simulink library "cdma2000_lib"  (Simulink 6.0)
settings: Solver=ode45  SolverMode=SingleTasking  StartTime=0.0  StopTime=10.0  RelTol=1e-3
values from neighbouring files (symbols this model uses):
  numTapsChEst = str2num(Vals{idxNumTapsChEst})    [wcdma_initmaskphlayer.m]    (also in wcdma_initmaskspreadandmod.m; wcdma_loadinitphlayer.m = 21; wcdma_loadinitspreadandmod.m = 21)
  overSampling = str2num(Vals{idxOverSampling})    [wcdma_initmaskphlayer.m]    (also in wcdma_initmaskspreadandmod.m; wcdma_loadinitphlayer.m = 8; wcdma_loadinitspreadandmod.m = 8)
undefined symbols (not defined in the file or in its folder): decPattern, gateRate, j, longCodeScrOff, magnitude, numPuncturedSymbols, numSymbPCGroup, overSamp, PCGroupInit, plcm_37, powerControlOff, qof_sign, scrBitRepetition, symbolTime, walshLength
libraries: dspsigops x30, dspsrcs4 x29, commutil2 x14, cdma2000_lib x13, commseqgen2 x10, dspbuff3 x9, dspsigattribs x7, dspindex x5, commsequence2 x4, commchan2 x3, simulink x3, dspmtrx3 x2
(part 1 of 2)
settings Model: Creator=arodrigu  LastModifiedBy=arodrigu  ProdHWDeviceType=Specified
settings DataIOCC: SignalLoggingName=logsOut
settings OptimizationCC: BooleanDataType=off
settings DebuggingCC: CheckExecutionContextPreStartOutputMsg=on  CheckExecutionContextRuntimeOutputMsg=on  SolverPrmCheckMsg=none
settings HardwareCC: ProdHWDeviceType=Specified  TargetUnknown=on
settings ModelReferenceCC: UpdateModelReferenceTargets=IfOutOfDate
settings SFSimCC: SFSimApplyToAllLibs=on  SFSimBuildMode=Incremental

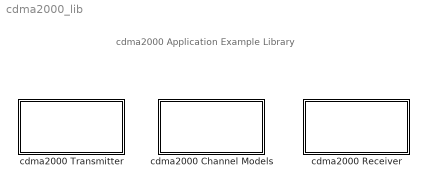
== system cdma2000_lib ==
  note: cdma2000 Application
      | Example Library
  cdma2000 Channel Models : Subsystem  PropExecContextAcrossSSBoundary=on
      mask Display: disp('cdma2000\nChannel Models')
  cdma2000 Receiver : Subsystem  PropExecContextAcrossSSBoundary=on
      mask Display: disp('cdma2000\nReceiver')
  cdma2000 Transmitter : Subsystem  PropExecContextAcrossSSBoundary=on
      mask Display: disp('cdma2000\nTransmitter')

== system cdma2000_lib/cdma2000 Channel Models ==
  note: cdma2000 Channel Models sublibrary
  AWGN Channel : Subsystem  PropExecContextAcrossSSBoundary=on  mask(cdma2000 Channel model: AWGN Channel){EsNodB=0}
      mask prompts: EsNodB "Es/No (dB):"
      mask Display: disp('AWGN Channel')
  Configurable Subsystem : Subsystem  BlockChoice=AWGN Channel  PropExecContextAcrossSSBoundary=on
      settings: TemplateBlock=self  MemberBlocks=AWGN Channel,Multipath Fading Channel,No Channel
  Multipath Fading Channel : Subsystem  PropExecContextAcrossSSBoundary=on  mask(cdma2000 Channel model: Multipath Fading Channel){EcN0=10, dopplerFreq=486, delayVector=[0 260e-9 521e-9 781e-9], gainVector=[0 -3 -6 -9]}
      mask prompts: EcN0 "EcN0 (in dB):"; dopplerFreq "Maximum Doppler Frequency shift (in Hz):"; delayVector "Multipath Profile - Delay Vector (s):"; gainVector "Multipath Profile - Gain Vector (dB):"
      mask Display: disp('Multipath Fading\nAWGN')
  No Channel : Subsystem  PropExecContextAcrossSSBoundary=on
      mask Type: cdma2000 Channel model: No Channel
      mask Display: disp('No Channel')

== system cdma2000_lib/cdma2000 Receiver ==
  note: cdma2000 Receiver sublibrary
  Channel Estimation : Subsystem  PropExecContextAcrossSSBoundary=on  mask(Channel Estimation){numTapsChEst=21}
      mask prompts: numTapsChEst "Number of Filter Taps for Channel Estimation:"
      mask help: Perform Channel Estimation
  Data Correlator : Subsystem  TreatAsAtomicUnit=on  PropExecContextAcrossSSBoundary=on
      mask Type: Data Correlator
  Long Code DeScrambling : Subsystem  PropExecContextAcrossSSBoundary=on
  Long Code DeScrambling Power Control Extracting : Subsystem  PropExecContextAcrossSSBoundary=on  mask(Long Code DeScrambling){radConfig=Radio Configuration 3, numSamp=768, nFrameMask=1, longCScrMask=Off, gateRateMask=1/4, TxDivMode=Non-TD, plcMask=[1 1 0 0 0 plcm_37]}
      mask prompts: radConfig "Radio Configuration:"; numSamp "Number of Samples per Frame:"; nFrameMask "Length of frame in multiples of 20 ms (n):"; longCScrMask "Long Code Scrambling"; gateRateMask "Gated Trasmission Rate:"; TxDivMode "Transmit Diversity Mode:"; plcMask "Public Long Code Mask:"
      mask help: Performs Long Code DeScrambling and Power Control Extraction for Forward Traffic Channel.
      mask init:
      | %-- Initialize parameters for Long Code Scrambling, Power Control
      | %-- and Signal Point Mapping
      | switch(get_param(gcb,'radConfig'))
      | 	case 'Radio Configuration 3'
      | 		Eb_PCCh = 1;
      | 		numPuncturedSymbols = 4;
      | 	% other cases
      | end	
      | 
      | %-- Transmit Diversity Mode
      | switch(TxDivMode)   
      |     case 1, % Non-Transmit Diversity
      |         decPattern = [47 46 45 44]+1; 
      |         scrBitRepetition = 1;    
      |     case {2,3} % Transmit Diversity: OTD, STS
      |         decPattern = [47 46 45]+1; 
      |         scrBitRepetition = 2;
      | end        
      | 
      | %-- Transmission Gating Rate
      | switch(gateRateMask)	
      | 	case 1 % No Power Control
      | 		powerControlOff = 0;
      | 		gateRate = 1;
      | 		PCGroupInit = 0;		
      |     case 2
      | 		powerControlOff = 1;
      |         gateRate = 1;
      |         PCGroupInit = 0;
      |     case 3
      | 		powerControlOff = 1;
      |         gateRate = 1/2;
      |         PCGroupInit = 0;
      |     case 4
      | 		powerControlOff = 1;
      |         gateRate = 1/4;
      |         PCGroupInit = 1;
      | end
      | 
      | %-- Long Code Scrambling
      | if(longCScrMask == 1)
      | 	longCodeScrOff = 0; % On
      | else
      | 	longCodeScrOff = 1; % Off
      | end
      | 
      | numSymbPCGroup = numSamp/((str2num(get_param(gcb,'nFrameMask')))*16);
      | symbolTime = 64/1.2288e6;
      mask Help: Performs Long Code DeScrambling and Power Control Extraction for Forward Traffic Channel.
      mask StyleString: popup(Radio Configuration 3),edit,popup(1|2|4),popup(On|Off),popup(Non Power Control|1|1/2|1/4),popup(Non-TD),edit
  Low Pass Filter : Subsystem  PropExecContextAcrossSSBoundary=on  mask(Low Pass Filter){N=21, Wn=1/4}
      mask prompts: N "Order of the Filter:"; Wn "Cut-off Frequency:"
      mask init:
      | h=fir1(N,Wn,kaiser(N+1,4))';
      mask Display: plot( 1:prod( size( h)), h);
  Rake Finger : Subsystem  TreatAsAtomicUnit=on  PropExecContextAcrossSSBoundary=on  mask(Rake Finger){walshLength=64, overSamp=4, chipRate=1.2288e6}
      mask prompts: walshLength "Forward Traffic Channel Walsh Length:"; overSamp "Oversampling Factor"; chipRate "Chip Rate"
      mask help: Each finger downsamples and decorrelates pilot bits and data using the corresponding sequence.
      mask init:
      | % Setting Sampling Time
      | st = walshLength/chipRate;
      mask Help: Each finger downsamples and decorrelates pilot bits and data using the corresponding sequence.
  Rake Receiver : Subsystem  PropExecContextAcrossSSBoundary=on  mask(Rake Receiver){walshLength=64, trChCode=63, pnOffset=0, qof_idx=0, numTapsChEst=11, numTapsRRC=48, overSampling=4, fingerEnables=[1 0 0 0], fingerPhases=[0 0 0 0]}
      mask prompts: walshLength "Forward Traffic Channel Walsh Length:"; trChCode "Forward Traffic Channel spreading code index:"; pnOffset "PN Sequence Offset (0..512):"; qof_idx "Quasi-orthogonal function index for F-DTCH:"; numTapsChEst "Number of Filter Taps for Channel Estimation:"; numTapsRRC "Number of Filter Taps for RRC filters:"; overSampling "Oversampling Factor:"; fingerEnables "Finger Enables:"; fingerPhases "Finger Phases (in units of Ticks):"
      mask help:
      | Rake receiver is made of 4 different fingers. Each finger downsamples and decorrelates pilot bits and data using the corresponding sequence.
      |
      | Pilot bits are then sent to the channel estimator whose output is then used to derotate the received data signal. The demodulated data processed by each rake finger is finally coherently combined.
      mask init:
      | %-- Sampling Time (corresponds to SF=64)
      | st =  walshLength/1.2288e6;
      | 
      | % Setting Parameters
      | numTapsRRC = numTapsRRC - (mod(numTapsRRC,2));
      | rxTicksDelay = numTapsRRC + fingerPhases;
      | 
      | %-- Quasi-orthogonal Function mask
      | qof_sign(1,:) = zeros(1,256);
      | qof_sign(2,:) = reshape(de2bi([hex2dec(['7228d7724eebebb1eb4eb1ebd78d8d28278282d81b41be1b411b1bbe7dd8277d']')'],'right-msb')',1,256);
      | qof_sign(3,:) = reshape(de2bi([hex2dec(['114b1e4444e14beeee4be144bbe1b4eedd872d77882d78dd2287d277772d87dd']')'],'right-msb')',1,256);
      | qof_sign(4,:) = reshape(de2bi([hex2dec(['1724bd71b28118d48ebddb172b187eb2e7d4b27ebd8ee82481b22be7dbe871bd']')'],'right-msb')',1,256);
      | 
      | %-- Walsh rotation
      | walshRotIdx = [0 130 173 47]+1;
      mask Help:
      | <p>Rake receiver is made of 4 different fingers. Each finger downsamples and decorrelates pilot bits and data using the corresponding sequence. </p>
      | 
      | <p>Pilot bits are then sent to the channel estimator whose output is then used to derotate the received data signal. The demodulated data processed by each rake finger is finally coherently combined.</p>
      mask StyleString: edit,edit,edit,popup(0|1|2|3),edit,edit,edit,edit,edit
  Rx Baseband Filtering : Subsystem  PropExecContextAcrossSSBoundary=on
      mask init:
      | % Load filter coefficients form MAT file
      | load cdma2000_rrcfil;
      | h_k = h_k/sqrt(4);
      mask Display: disp('RC Filter')
  Rx Channel Structure : Subsystem  PropExecContextAcrossSSBoundary=on
  Symbol Demapping : Subsystem  PropExecContextAcrossSSBoundary=on
      mask Display: disp('Symbol\nDemapping');

== system cdma2000_lib/cdma2000 Transmitter ==
  note: cdma2000 Transmitter sublibrary
  Baseband Filtering : Subsystem  PropExecContextAcrossSSBoundary=on
      mask init:
      | % Load filter coefficients form MAT file
      | load cdma2000_rrcfil;
      mask Display: disp('RC Filter')
  Long Code Scrambling : Subsystem  PropExecContextAcrossSSBoundary=on
  Long Code Scrambling Power Control and Signal Point Mapping : Subsystem  PropExecContextAcrossSSBoundary=on  mask(Long Code Scrambling){radConfig=Radio Configuration 3, numSamp=768, nFrameMask=1, longCScrMask=Off, gateRateMask=1/4, TxDivMode=Non-TD, plcMask=[1 1 0 0 0 plcm_37]}
      mask prompts: radConfig "Radio Configuration:"; numSamp "Number of Samples per Frame:"; nFrameMask "Length of frame in multiples of 20 ms (n):"; longCScrMask "Long Code Scrambling"; gateRateMask "Gated Trasmission Rate:"; TxDivMode "Transmit Diversity Mode:"; plcMask "Public Long Code Mask:"
      mask help: Performs Long Code Scrambling, Power Control and Signal Point Mapping for Forward Traffic Channel.
      mask init:
      | %-- Initialize parameters for Long Code Scrambling, Power Control
      | %-- and Signal Point Mapping
      | 
      | switch(get_param(gcb,'radConfig'))
      | 	case 'Radio Configuration 3'
      | 		Eb_PCCh = 1;
      | 		numPuncturedSymbols = 4;
      | 	% other cases
      | end	
      | 
      | %-- Transmit Diversity Mode
      | switch(TxDivMode)   
      |     case 1, % Non-Transmit Diversity
      |         decPattern = [47 46 45 44]+1; 
      |         scrBitRepetition = 1;    
      |     case {2,3} % Transmit Diversity: OTD, STS
      |         decPattern = [47 46 45]+1; 
      |         scrBitRepetition = 2;
      | end        
      | 
      | %-- Transmission Gating Rate
      | 
      | switch(gateRateMask)	
      | 	case 1 % No Power Control
      | 		powerControlOff = 0;
      | 		gateRate = 1;
      | 		PCGroupInit = 0;		
      |     case 2
      | 		powerControlOff = 1;
      |         gateRate = 1;
      |         PCGroupInit = 0;
      |     case 3
      | 		powerControlOff = 1;
      |         gateRate = 1/2;
      |         PCGroupInit = 0;
      |     case 4
      | 		powerControlOff = 1;
      |         gateRate = 1/4;
      |         PCGroupInit = 1;
      | end
      | 
      | %-- Long Code Scrambling
      | if(longCScrMask == 1)
      | 	longCodeScrOff = 0; % On
      | else
      | 	longCodeScrOff = 1; % Off
      | end
      | 
      | numSymbPCGroup = numSamp/((str2num(get_param(gcb,'nFrameMask')))*16);
      | symbolTime = 64/1.2288e6;
      mask Help: Performs Long Code Scrambling, Power Control and Signal Point Mapping for Forward Traffic Channel.
      mask StyleString: popup(Radio Configuration 3),edit,popup(1|2|4),popup(On|Off),popup(Non Power Control|1|1/2|1/4),popup(Non-TD),edit
  Non-TD Demultiplexer : Subsystem  PropExecContextAcrossSSBoundary=on
      mask Type: Non-TD Demultiplexer
      mask Description: Outputs first input symbol of the frame to the I1 and the subsequent symbols to Q1,I1, .. outputs as described in 3.1.3.1.11.1
      mask Help: Outputs first input symbol of the frame to the I1 and the subsequent symbols to Q1,I1, .. outputs ase described in 3.1.3.1.11.1
  Power Control Bit Position Extractor : Subsystem  PropExecContextAcrossSSBoundary=on
  Power Control Symbol Puncture : Subsystem  PropExecContextAcrossSSBoundary=on
  Spreading Non-TD Mode : Subsystem  PropExecContextAcrossSSBoundary=on  mask(Spreading Non-TD Mode){walshLength=64, trChCode=63, qof_idx=0, pnOffset=0}
      mask prompts: walshLength "Forward Traffic Channel Walsh Length:"; trChCode "Forward Traffic Channel spreading code index:"; qof_idx "Quasi-orthogonal function index for F-DTCH:"; pnOffset "PN Sequence Offset (0..512):"
      mask help: Performs Orthogonal spreading using a real-valued Quasi-Orthogonal function and Quadrature spreading using a complex-valued PN sequence as described in 3.1.3.1.12
      mask init:
      | %-- Quasi-orthogonal Function mask
      | qof_sign(1,:) = zeros(1,256);
      | qof_sign(2,:) = reshape(de2bi([hex2dec(['7228d7724eebebb1eb4eb1ebd78d8d28278282d81b41be1b411b1bbe7dd8277d']')'],'right-msb')',1,256);
      | qof_sign(3,:) = reshape(de2bi([hex2dec(['114b1e4444e14beeee4be144bbe1b4eedd872d77882d78dd2287d277772d87dd']')'],'right-msb')',1,256);
      | qof_sign(4,:) = reshape(de2bi([hex2dec(['1724bd71b28118d48ebddb172b187eb2e7d4b27ebd8ee82481b22be7dbe871bd']')'],'right-msb')',1,256);
      | 
      | %-- Walsh rotation
      | walshRotIdx = [0 130 173 47]+1;
      mask Help: Performs Orthogonal spreading using a real-valued Quasi-Orthogonal function and Quadrature spreading using a complex-valued PN sequence as described in 3.1.3.1.12
      mask StyleString: edit,edit,popup(0|1|2|3),edit
  Tx Channel Structure : Subsystem  PropExecContextAcrossSSBoundary=on

== system cdma2000_lib/cdma2000 Channel Models/AWGN Channel ==
  In1 : Inport  LatchInput=off
  AWGN Channel : commchan2/AWGN Channel  seed=67  noiseMode="Signal to noise ratio  (Es/No)"  EbNodB=10  EsNodB=EsNodB  SNRdB=10  bitsPerSym=1  Ps=1  Tsym=1/1.2288e6  variance=1
  Out1 : Outport
  wires:
  In1/1 -> AWGN Channel/1
  AWGN Channel/1 -> Out1/1

== system cdma2000_lib/cdma2000 Channel Models/Configurable Subsystem ==
  In1 : Inport  LatchInput=off
  AWGN Channel : cdma2000_lib/cdma2000 Channel Models/AWGN Channel  EsNodB=0
  Out1 : Outport
  wires:
  In1/1 -> AWGN Channel/1
  AWGN Channel/1 -> Out1/1

== system cdma2000_lib/cdma2000 Channel Models/Multipath Fading Channel ==
  In1 : Inport  LatchInput=off
  AWGN Channel : commchan2/AWGN Channel  seed=67  noiseMode="Signal to noise ratio  (Es/No)"  EbNodB=10  EsNodB=EcN0  SNRdB=10  bitsPerSym=1  Ps=1  Tsym=1/1.2288e6  variance=1
  Multipath Rayleigh Fading Channel : commchan2/Multipath Rayleigh Fading Channel  Fd=dopplerFreq  simTs=1/(1.2288e6*4)  delayVec=delayVector  gainVecdB=gainVector  normGain=off  Seed=73
  Out1 : Outport
  wires:
  Multipath Rayleigh Fading Channel/1 -> AWGN Channel/1
  AWGN Channel/1 -> Out1/1
  In1/1 -> Multipath Rayleigh Fading Channel/1

== system cdma2000_lib/cdma2000 Channel Models/No Channel ==
  In1 : Inport  LatchInput=off
  Out1 : Outport
  wires:
  In1/1 -> Out1/1

== system cdma2000_lib/cdma2000 Receiver/Channel Estimation ==
  note: Channel Estimation
  cRef : Inport  LatchInput=off
  cRx : Inport  Port=2  LatchInput=off
  Low Pass Filter : cdma2000_lib/cdma2000 Receiver/Low Pass Filter  N=numTapsChEst-1  Wn=1/4
  Math Function : Math  Operator=conj  OutputSignalType=complex  SaturateOnIntegerOverflow=on
  Product : Product  SaturateOnIntegerOverflow=on  InputSameDT=on
  chEst : Outport
  wires:
  cRef/1 -> Math Function/1  "Ref"
  Math Function/1 -> Product/1
  Product/1 -> Low Pass Filter/1  "noisy channel estimate"
  cRx/1 -> Product/2  "Output of  Pilot Correlator"
  Low Pass Filter/1 -> chEst/1  "channel estimate"

== system cdma2000_lib/cdma2000 Receiver/Data Correlator ==
  note: Chip Correlator
  cIn : Inport  LatchInput=off
  cPNseq : Inport  Port=2  LatchInput=off
  Enable : EnablePort
  Downsample : dspsigops/Downsample  N=overSamp  phase=0  ic=0  smode=Force single rate  fmode=Maintain input frame rate
  Gain : Gain  Gain=1/walshLength  SaturateOnIntegerOverflow=on
  Integrate and Dump : commfilt2/Integrate and Dump  obssamples=walshLength  offsetsamples=0  nodump=off
  Math Function : Math  Operator=conj  OutputSignalType=complex  SaturateOnIntegerOverflow=on
  Product2 : Product  Inputs=**  SaturateOnIntegerOverflow=on  InputSameDT=on
  cOutBits : Outport
  wires:
  Math Function/1 -> Product2/2
  cPNseq/1 -> Math Function/1  "Chips Code"
  cIn/1 -> Downsample/1  "Ticks Signal"
  Downsample/1 -> Product2/1  "Chip Signal"
  Product2/1 -> Integrate and Dump/1  "Correlation"
  Integrate and Dump/1 -> Gain/1
  Gain/1 -> cOutBits/1

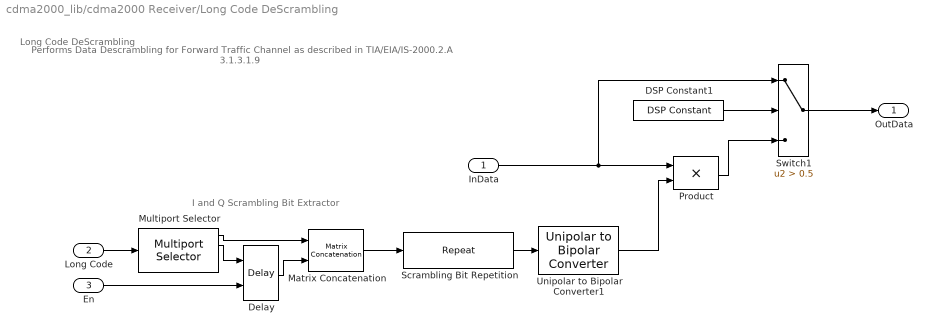
== system cdma2000_lib/cdma2000 Receiver/Long Code DeScrambling ==
  note: I and Q Scrambling Bit Extractor
  note: Long Code DeScrambling
  note: Performs Data Descrambling for Forward Traffic Channel as described in TIA/EIA/IS-2000.2.A 3.1.3.1.9
  InData : Inport  LatchInput=off
  Long Code : Inport  Port=2  LatchInput=off
  En : Inport  Port=3  LatchInput=off
  DSP Constant1 : dspsrcs4/DSP Constant  Value=longCodeScrOff  SampleMode=Discrete  discreteOutput=Sample-based  continuousOutput=Sample-based  sampTime=symbolTime*scrBitRepetition  framePeriod=symbolTime*scrBitRepetition  dataType=Inherit from 'Constant value'  wordLen=16  udDataType=sfix(16)  fracBitsMode=Best precision  numFracBits=15  InterpretAs1D=off  Ts=symbolTime*scrBitRepetition  FramebasedOutput=off
      settings: AttributesFormatString=\n\n\n\n
  Delay : dspsigops/Delay  dly_unit=Samples  delay=1  ic_detail=on  dif_ic_for_ch=off  dif_ic_for_dly=off  ic=0  reset_popup=Rising edge
  Matrix Concatenation : simulink/Math Operations/Matrix Concatenation  numInports=2  catMethod=Vertical
  Multiport Selector : dspindex/Multiport Selector  rowsOrCols=Rows  idxCellArray={ 1,64*scrBitRepetition}  idxErrMode=Clip Index
      settings: AttributesFormatString=\n
  Product : Product  SaturateOnIntegerOverflow=on
  Scrambling Bit Repetition : dspsigops/Repeat  N=scrBitRepetition  ic=0  mode=Maintain input frame rate
  Switch1 : Switch  Criteria=u2 > Threshold  Threshold=0.5  SaturateOnIntegerOverflow=on
  Unipolar to Bipolar Converter1 : commutil2/Unipolar to Bipolar Converter  M=2  polarity=Negative
  OutData : Outport
  wires:
  Long Code/1 -> Multiport Selector/1
  Multiport Selector/1 -> Matrix Concatenation/1
  Multiport Selector/2 -> Delay/1
  Delay/1 -> Matrix Concatenation/2
  Matrix Concatenation/1 -> Scrambling Bit Repetition/1
  Scrambling Bit Repetition/1 -> Unipolar to Bipolar Converter1/1
  Unipolar to Bipolar Converter1/1 -> Product/2
  InData/1 -> Product/1, Switch1/1
  DSP Constant1/1 -> Switch1/2
  Product/1 -> Switch1/3
  Switch1/1 -> OutData/1
  En/1 -> Delay/2

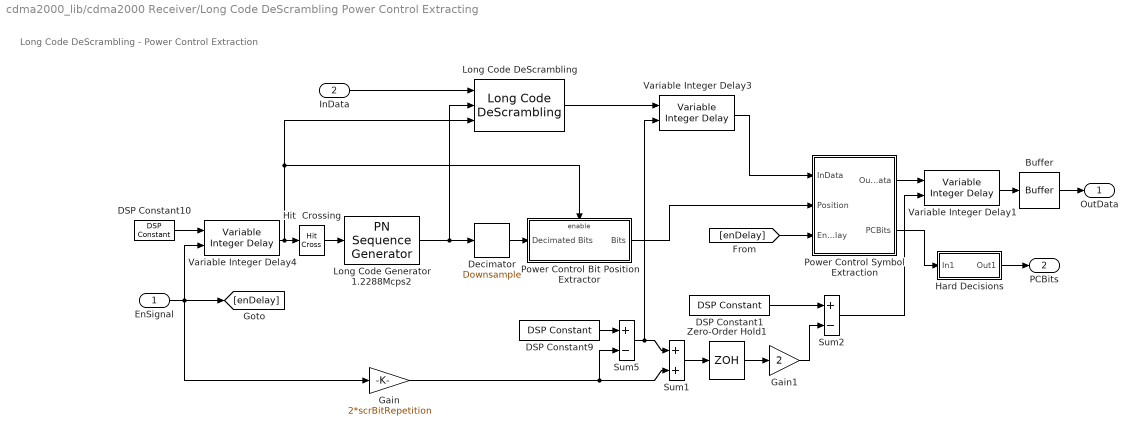
== system cdma2000_lib/cdma2000 Receiver/Long Code DeScrambling Power Control Extracting ==
  note: Long Code DeScrambling - Power Control Extraction
  EnSignal : Inport  LatchInput=off
  InData : Inport  Port=2  LatchInput=off
  Buffer : dspbuff3/Buffer  N=numSamp  V=0  ic=0
  DSP Constant1 : dspsrcs4/DSP Constant  Value=numSamp  SampleMode=Discrete  discreteOutput=Sample-based  continuousOutput=Sample-based  sampTime=20e-3/16  framePeriod=20e-3/16  dataType=Inherit from 'Constant value'  wordLen=16  udDataType=sfix(16)  fracBitsMode=Best precision  numFracBits=15  InterpretAs1D=off  Ts=20e-3/16  FramebasedOutput=off
  DSP Constant10 : dspsrcs4/DSP Constant  Value=1  SampleMode=Discrete  discreteOutput=Sample-based  continuousOutput=Sample-based  sampTime=64/1.2288e6  framePeriod=64/1.2288e6  dataType=Inherit from 'Constant value'  wordLen=16  udDataType=sfix(16)  fracBitsMode=Best precision  numFracBits=15  InterpretAs1D=off  Ts=64/1.2288e6  FramebasedOutput=off
  DSP Constant9 : dspsrcs4/DSP Constant  Value=numSamp/16  SampleMode=Discrete  discreteOutput=Sample-based  continuousOutput=Sample-based  sampTime=64/1.2288e6  framePeriod=64/1.2288e6  dataType=Inherit from 'Constant value'  wordLen=16  udDataType=sfix(16)  fracBitsMode=Best precision  numFracBits=15  InterpretAs1D=off  Ts=64/1.2288e6  FramebasedOutput=off
  Decimator : dspsigops/Downsample  N=64/2  phase=0  ic=0  smode=Allow multirate  fmode=Maintain input frame rate
      settings: AttributesFormatString=\n
  Gain : Gain  Gain=2*scrBitRepetition  SaturateOnIntegerOverflow=on
  Gain1 : Gain  Gain=2  SaturateOnIntegerOverflow=on
  Hard Decisions : Subsystem  PropExecContextAcrossSSBoundary=on
      mask Display: disp('Hard\nDecisions');
  Hit  Crossing : HitCross  HitCrossingOffset=0.5  HitCrossingDirection=rising  ZeroCross=off
  Long Code DeScrambling : cdma2000_lib/cdma2000 Receiver/Long Code DeScrambling  SimViewingDevice=off  DataTypeOverride=UseLocalSettings  MinMaxOverflowLogging=UseLocalSettings
      settings: Permissions=ReadWrite  RTWFcnNameOpts=Auto  RTWFileNameOpts=Auto
  Long Code Generator 1.2288Mcps2 : commseqgen2/PN Sequence Generator  poly=[42 35 33 31 27 26 25 22 21 19 18 17 16 10 7 6 5 3 2 1 0]  ini_sta=[1]  shift=plcMask  Ts=1/1.2288e6  frameBased=on  sampPerFrame=64*scrBitRepetition  reset=on
  Power Control Bit Position Extractor : Subsystem  PropExecContextAcrossSSBoundary=on
  Power Control Symbol Extraction : Subsystem  PropExecContextAcrossSSBoundary=on
  Sum1 : Sum  SaturateOnIntegerOverflow=on
  Sum2 : Sum  Inputs=+-  SaturateOnIntegerOverflow=on
  Sum5 : Sum  Inputs=+-  SaturateOnIntegerOverflow=on
  Variable Integer Delay1 : dspsigops/Variable Integer Delay  dmax=numSamp+10  ic=0
  Variable Integer Delay3 : dspsigops/Variable Integer Delay  dmax=numSamp+10  ic=0
  Variable Integer Delay4 : dspsigops/Variable Integer Delay  dmax=100  ic=0
  Zero-Order Hold1 : ZeroOrderHold  SampleTime=20e-3/16
  OutData : Outport
  PCBits : Outport  Port=2
  wires:
  [enDelay] -> Power Control Symbol Extraction/3(EnDelay)
  Zero-Order Hold1/1 -> Gain1/1
  Hard Decisions/1(Out1) -> PCBits/1
  Gain1/1 -> Sum2/2
  DSP Constant1/1 -> Sum2/1
  Sum1/1 -> Zero-Order Hold1/1
  Sum2/1 -> Variable Integer Delay1/2
  Power Control Symbol Extraction/2(PCBits) -> Hard Decisions/1(In1)
  Power Control Symbol Extraction/1(OutData) -> Variable Integer Delay1/1
  Long Code DeScrambling/1 -> Variable Integer Delay3/1
  Sum5/1 -> Sum1/1, Variable Integer Delay3/2
  Variable Integer Delay3/1 -> Power Control Symbol Extraction/1(InData)
  Power Control Bit Position Extractor/1(Bits) -> Power Control Symbol Extraction/2(Position)
  Buffer/1 -> OutData/1
  Gain/1 -> Sum1/2, Sum5/2
  DSP Constant9/1 -> Sum5/1
  Variable Integer Delay1/1 -> Buffer/1
  DSP Constant10/1 -> Variable Integer Delay4/1
  EnSignal/1 -> [enDelay], Gain/1, Variable Integer Delay4/2
  Variable Integer Delay4/1 -> Power Control Bit Position Extractor/Enable, Long Code DeScrambling/3, Hit  Crossing/1
  Hit  Crossing/1 -> Long Code Generator 1.2288Mcps2/1
  InData/1 -> Long Code DeScrambling/1
  Decimator/1 -> Power Control Bit Position Extractor/1(Decimated Bits)
  Long Code Generator 1.2288Mcps2/1 -> Long Code DeScrambling/2, Decimator/1

== system cdma2000_lib/cdma2000 Receiver/Low Pass Filter ==
  In1 : Inport  LatchInput=off
  Digital Filter : dsparch4/Digital Filter  TypePopup=FIR (all zeros)  IIRFiltStruct=Direct form II transposed  AllPoleFiltStruct=Direct form  FIRFiltStruct=Direct form  CoeffSource=Specify via dialog  NumCoeffs=h  DenCoeffs=[1 0.1]  BiQuadCoeffs=[1 0.3 0.4 1 0.1 0.2]  LatticeCoeffs=[0.2 0.4]  denIgnore=on  FiltPerSampPopup=One filter per frame  IC=0  ICnum=0  ICden=0  roundingMode=Floor  overflowMode=off
  Out1 : Outport
  wires:
  In1/1 -> Digital Filter/1
  Digital Filter/1 -> Out1/1

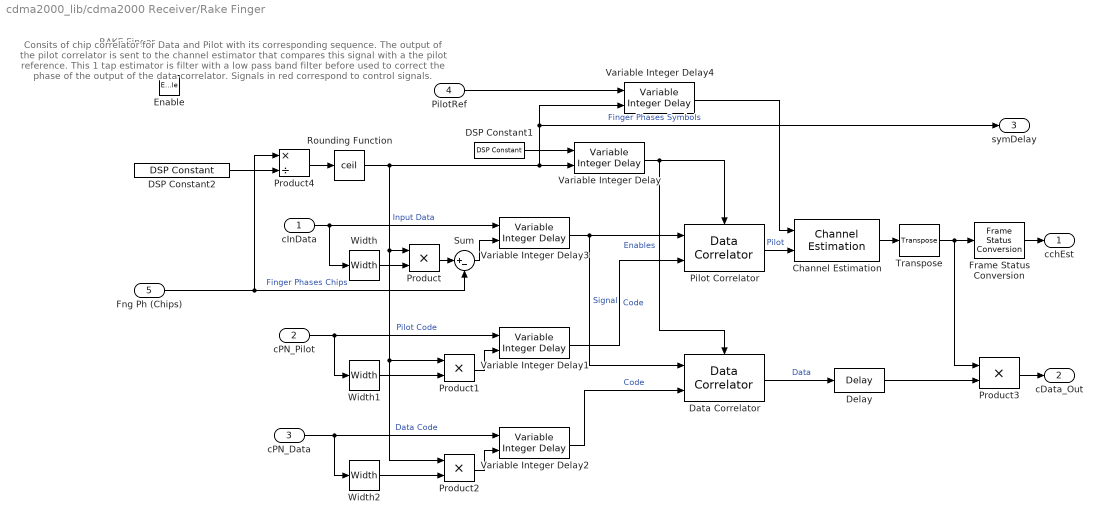
== system cdma2000_lib/cdma2000 Receiver/Rake Finger ==
  note: RAKE Finger
  note: Consits of chip correlator for Data and Pilot with its corresponding sequence. The output of the pilot correlator is sent to the channel estimator that compares this signal
      | with a the pilot reference. This 1 tap estimator is filter with a low pass band filter before used to correct the phase of the output of the data correlator.
      | Signals in red correspond to control signals.
  cInData : Inport  LatchInput=off
  cPN_Pilot : Inport  Port=2  LatchInput=off
  cPN_Data : Inport  Port=3  LatchInput=off
  PilotRef : Inport  Port=4  LatchInput=off
  Fng Ph (Chips) : Inport  Port=5  LatchInput=off
  Enable : EnablePort
  Channel Estimation : cdma2000_lib/cdma2000 Receiver/Channel Estimation  numTapsChEst=numTapsChEst
  DSP Constant1 : dspsrcs4/DSP Constant  Value=1  SampleMode=Discrete  discreteOutput=Sample-based  continuousOutput=Sample-based  sampTime=st  framePeriod=st  dataType=Inherit from 'Constant value'  wordLen=16  udDataType=sfix(16)  fracBitsMode=Best precision  numFracBits=15  InterpretAs1D=off  Ts=st  FramebasedOutput=off
  DSP Constant2 : dspsrcs4/DSP Constant  Value=overSampling*walshLength  SampleMode=Discrete  discreteOutput=Sample-based  continuousOutput=Sample-based  sampTime=st  framePeriod=st  dataType=Inherit from 'Constant value'  wordLen=16  udDataType=sfix(16)  fracBitsMode=Best precision  numFracBits=15  InterpretAs1D=off  Ts=st  FramebasedOutput=off
  Data Correlator : cdma2000_lib/cdma2000 Receiver/Data Correlator
  Delay : dspsigops/Delay  dly_unit=Samples  delay=((numTapsChEst-1)/2)  ic_detail=off  dif_ic_for_ch=off  dif_ic_for_dly=off  ic=0  reset_popup=None
  Frame Status Conversion : dspsigattribs/Frame Status Conversion  growRefPort=off  outframe=Frame-based
  Pilot Correlator : cdma2000_lib/cdma2000 Receiver/Data Correlator
  Product{,1..3} (4 alike) : Product  SaturateOnIntegerOverflow=on  InputSameDT=on
  Product4 : Product  Inputs=*/  SaturateOnIntegerOverflow=on  InputSameDT=on
  Rounding Function : Rounding  Operator=ceil
  Sum : Sum  Inputs=|+-  SaturateOnIntegerOverflow=on  InputSameDT=on
  Transpose : dspmtrx3/Transpose  Hermitian=on  overflowFlag=on
  Variable Integer Delay : dspsigops/Variable Integer Delay  dmax=100  ic=0
  Variable Integer Delay1 : dspsigops/Variable Integer Delay  dmax=20*walshLength*overSampling  ic=0
  Variable Integer Delay2 : dspsigops/Variable Integer Delay  dmax=20*walshLength*overSampling  ic=0
  Variable Integer Delay3 : dspsigops/Variable Integer Delay  dmax=20*walshLength*overSampling  ic=0
  Variable Integer Delay4 : dspsigops/Variable Integer Delay  dmax=20  ic=0
  Width : Width
  Width1 : Width
  Width2 : Width
  cchEst : Outport
  cData_Out : Outport  Port=2
  symDelay : Outport  Port=3
  wires:
  Frame Status Conversion/1 -> cchEst/1
  DSP Constant2/1 -> Product4/2
  Product4/1 -> Rounding Function/1
  Variable Integer Delay2/1 -> Data Correlator/2  "Code"
  Fng Ph (Chips)/1 -> Product4/1, Sum/2  "Finger Phases Chips"
  Sum/1 -> Variable Integer Delay3/2
  Product/1 -> Sum/1
  Width2/1 -> Product2/2
  Product2/1 -> Variable Integer Delay2/2
  cPN_Data/1 -> Variable Integer Delay2/1, Width2/1  "Data Code"
  Width1/1 -> Product1/2
  Width/1 -> Product/2
  Product1/1 -> Variable Integer Delay1/2
  Rounding Function/1 -> Product/1, Product1/1, Product2/1, Variable Integer Delay/2, Variable Integer Delay4/2, symDelay/1  "Finger Phases Symbols"
  cInData/1 -> Width/1, Variable Integer Delay3/1  "Input Data"
  Variable Integer Delay3/1 -> Pilot Correlator/1, Data Correlator/1  "Signal"
  Data Correlator/1 -> Delay/1  "Data"
  Variable Integer Delay/1 -> Pilot Correlator/Enable, Data Correlator/Enable  "Enables"
  DSP Constant1/1 -> Variable Integer Delay/1
  cPN_Pilot/1 -> Width1/1, Variable Integer Delay1/1  "Pilot Code"
  Variable Integer Delay1/1 -> Pilot Correlator/2  "Code"
  Pilot Correlator/1 -> Channel Estimation/2  "Pilot"
  Channel Estimation/1 -> Transpose/1
  Delay/1 -> Product3/2
  Transpose/1 -> Frame Status Conversion/1, Product3/1
  Product3/1 -> cData_Out/1
  PilotRef/1 -> Variable Integer Delay4/1
  Variable Integer Delay4/1 -> Channel Estimation/1

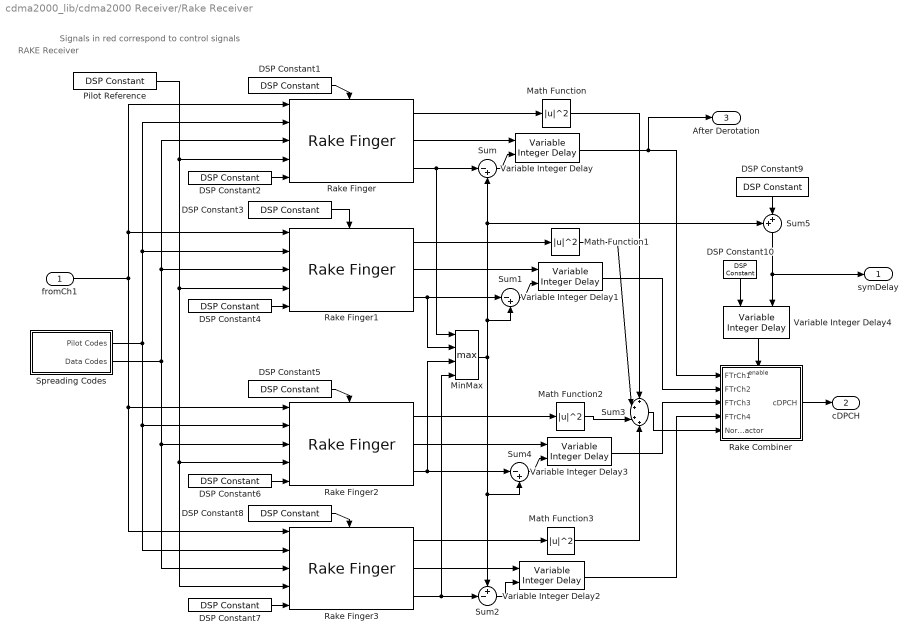
== system cdma2000_lib/cdma2000 Receiver/Rake Receiver ==
  note: RAKE Receiver
  note: Signals in red correspond to control signals
  fromCh1 : Inport  LatchInput=off
  DSP Constant1 : dspsrcs4/DSP Constant  Value=fingerEnables(1)  SampleMode=Discrete  discreteOutput=Sample-based  continuousOutput=Sample-based  sampTime=st  framePeriod=st  dataType=Inherit from 'Constant value'  wordLen=16  udDataType=sfix(16)  fracBitsMode=Best precision  numFracBits=15  InterpretAs1D=off  Ts=st  FramebasedOutput=off
  DSP Constant10 : dspsrcs4/DSP Constant  Orientation=down  Value=1  SampleMode=Discrete  discreteOutput=Sample-based  continuousOutput=Sample-based  sampTime=st  framePeriod=st  dataType=Inherit from 'Constant value'  wordLen=16  udDataType=sfix(16)  fracBitsMode=Best precision  numFracBits=15  InterpretAs1D=off  Ts=st  FramebasedOutput=off
  DSP Constant2 : dspsrcs4/DSP Constant  Value=rxTicksDelay(1)  SampleMode=Discrete  discreteOutput=Sample-based  continuousOutput=Sample-based  sampTime=st  framePeriod=st  dataType=Inherit from 'Constant value'  wordLen=16  udDataType=sfix(16)  fracBitsMode=Best precision  numFracBits=15  InterpretAs1D=off  Ts=st  FramebasedOutput=off
  DSP Constant3 : dspsrcs4/DSP Constant  Value=fingerEnables(2)  SampleMode=Discrete  discreteOutput=Sample-based  continuousOutput=Sample-based  sampTime=st  framePeriod=st  dataType=Inherit from 'Constant value'  wordLen=16  udDataType=sfix(16)  fracBitsMode=Best precision  numFracBits=15  InterpretAs1D=off  Ts=st  FramebasedOutput=off
  DSP Constant4 : dspsrcs4/DSP Constant  Value=rxTicksDelay(2)  SampleMode=Discrete  discreteOutput=Sample-based  continuousOutput=Sample-based  sampTime=st  framePeriod=st  dataType=Inherit from 'Constant value'  wordLen=16  udDataType=sfix(16)  fracBitsMode=Best precision  numFracBits=15  InterpretAs1D=off  Ts=st  FramebasedOutput=off
  DSP Constant5 : dspsrcs4/DSP Constant  Value=fingerEnables(3)  SampleMode=Discrete  discreteOutput=Sample-based  continuousOutput=Sample-based  sampTime=st  framePeriod=st  dataType=Inherit from 'Constant value'  wordLen=16  udDataType=sfix(16)  fracBitsMode=Best precision  numFracBits=15  InterpretAs1D=off  Ts=st  FramebasedOutput=off
  DSP Constant6 : dspsrcs4/DSP Constant  Value=rxTicksDelay(3)  SampleMode=Discrete  discreteOutput=Sample-based  continuousOutput=Sample-based  sampTime=st  framePeriod=st  dataType=Inherit from 'Constant value'  wordLen=16  udDataType=sfix(16)  fracBitsMode=Best precision  numFracBits=15  InterpretAs1D=off  Ts=st  FramebasedOutput=off
  DSP Constant7 : dspsrcs4/DSP Constant  Value=rxTicksDelay(4)  SampleMode=Discrete  discreteOutput=Sample-based  continuousOutput=Sample-based  sampTime=st  framePeriod=st  dataType=Inherit from 'Constant value'  wordLen=16  udDataType=sfix(16)  fracBitsMode=Best precision  numFracBits=15  InterpretAs1D=off  Ts=st  FramebasedOutput=off
  DSP Constant8 : dspsrcs4/DSP Constant  Value=fingerEnables(4)  SampleMode=Discrete  discreteOutput=Sample-based  continuousOutput=Sample-based  sampTime=st  framePeriod=st  dataType=Inherit from 'Constant value'  wordLen=16  udDataType=sfix(16)  fracBitsMode=Best precision  numFracBits=15  InterpretAs1D=off  Ts=st  FramebasedOutput=off
  DSP Constant9 : dspsrcs4/DSP Constant  Orientation=down  Value=((numTapsChEst-1)/2)  SampleMode=Discrete  discreteOutput=Sample-based  continuousOutput=Sample-based  sampTime=st  framePeriod=st  dataType=Inherit from 'Constant value'  wordLen=16  udDataType=sfix(16)  fracBitsMode=Best precision  numFracBits=15  InterpretAs1D=off  Ts=st  FramebasedOutput=off
  Math Function{,1..3} (4 alike) : Math  Operator=magnitude^2  SaturateOnIntegerOverflow=on
  MinMax : MinMax  Function=max  Inputs=4  SaturateOnIntegerOverflow=on  InputSameDT=on
  Pilot Reference : dspsrcs4/DSP Constant  Value=1  SampleMode=Discrete  discreteOutput=Frame-based  continuousOutput=Sample-based  sampTime=64/1.2288e6  framePeriod=64/1.2288e6  dataType=Inherit from 'Constant value'  wordLen=16  udDataType=sfix(16)  fracBitsMode=Best precision  numFracBits=15  InterpretAs1D=off  Ts=64/1.2288e6  FramebasedOutput=on
  Rake Combiner : Subsystem  TreatAsAtomicUnit=on  PropExecContextAcrossSSBoundary=on
      mask Type: Rake Combiner
      mask Description: Performs Rake combjner by averaging the output of enabled Rake Fingers blocks.
  Rake Finger{,1..3} (4 alike) : cdma2000_lib/cdma2000 Receiver/Rake Finger  walshLength=64  overSamp=4  chipRate=1.2288e6
  Spreading Codes : Subsystem  PropExecContextAcrossSSBoundary=on
  Sum : Sum  Inputs=|-+  SaturateOnIntegerOverflow=on
  Sum1 : Sum  Inputs=|-+  SaturateOnIntegerOverflow=on
  Sum2 : Sum  Inputs=+-|  SaturateOnIntegerOverflow=on
  Sum3 : Sum  Inputs=++++  SaturateOnIntegerOverflow=on  InputSameDT=on
  Sum4 : Sum  Inputs=|-+  SaturateOnIntegerOverflow=on
  Sum5 : Sum  Orientation=down  Inputs=++|  SaturateOnIntegerOverflow=on
  Variable Integer Delay{,1..3} (4 alike) : dspsigops/Variable Integer Delay  dmax=100  ic=0
  Variable Integer Delay4 : dspsigops/Variable Integer Delay  Orientation=down  dmax=100  ic=0
  symDelay : Outport
  cDPCH : Outport  Port=2
  After Derotation : Outport  Port=3
  wires:
  DSP Constant9/1 -> Sum5/2
  Variable Integer Delay2/1 -> Rake Combiner/4(FTrCh4)
  Variable Integer Delay3/1 -> Rake Combiner/3(FTrCh3)
  Variable Integer Delay1/1 -> Rake Combiner/2(FTrCh2)
  Variable Integer Delay/1 -> Rake Combiner/1(FTrCh1), After Derotation/1
  Math Function3/1 -> Sum3/4
  Rake Finger3/1 -> Math Function3/1
  Math Function2/1 -> Sum3/3
  Rake Finger2/1 -> Math Function2/1
  Math Function1/1 -> Sum3/2
  Rake Finger1/1 -> Math Function1/1
  Rake Combiner/1(cDPCH) -> cDPCH/1
  Sum3/1 -> Rake Combiner/5(Norm Factor)
  Sum4/1 -> Variable Integer Delay3/2
  Rake Finger2/2 -> Variable Integer Delay3/1
  Sum2/1 -> Variable Integer Delay2/2
  Rake Finger3/2 -> Variable Integer Delay2/1
  Rake Finger1/2 -> Variable Integer Delay1/1
  Sum1/1 -> Variable Integer Delay1/2
  Sum/1 -> Variable Integer Delay/2
  MinMax/1 -> Sum4/2, Sum2/1, Sum1/2, Sum/2, Sum5/1
  Rake Finger3/3 -> Sum2/2, MinMax/4
  Rake Finger2/3 -> Sum4/1, MinMax/3
  Rake Finger1/3 -> Sum1/1, MinMax/2
  Rake Finger/3 -> Sum/1, MinMax/1
  DSP Constant7/1 -> Rake Finger3/5
  DSP Constant8/1 -> Rake Finger3/Enable
  DSP Constant6/1 -> Rake Finger2/5
  DSP Constant5/1 -> Rake Finger2/Enable
  DSP Constant4/1 -> Rake Finger1/5
  DSP Constant3/1 -> Rake Finger1/Enable
  fromCh1/1 -> Rake Finger2/1, Rake Finger3/1, Rake Finger1/1, Rake Finger/1
  DSP Constant1/1 -> Rake Finger/Enable
  Rake Finger/2 -> Variable Integer Delay/1
  Rake Finger/1 -> Math Function/1
  DSP Constant2/1 -> Rake Finger/5
  Spreading Codes/1(Pilot Codes) -> Rake Finger2/2, Rake Finger3/2, Rake Finger1/2, Rake Finger/2
  Spreading Codes/2(Data Codes) -> Rake Finger2/3, Rake Finger3/3, Rake Finger1/3, Rake Finger/3
  Pilot Reference/1 -> Rake Finger2/4, Rake Finger3/4, Rake Finger1/4, Rake Finger/4
  Math Function/1 -> Sum3/1
  Sum5/1 -> Variable Integer Delay4/2, symDelay/1
  DSP Constant10/1 -> Variable Integer Delay4/1
  Variable Integer Delay4/1 -> Rake Combiner/Enable

== system cdma2000_lib/cdma2000 Receiver/Rx Baseband Filtering ==
  note: Baseband Filtering
  note: I and Q components are applied to the I and Q baseband filters separately
      | as described in 3.1.3.1.12
  InData : Inport  LatchInput=off
  Filtering : dspmlti3/FIR Interpolation  h=h_k  L=1  framing=Maintain input frame rate  outputBufInitCond=0  roundingMode=Floor  overflowMode=off
  OutData : Outport
  wires:
  Filtering/1 -> OutData/1
  InData/1 -> Filtering/1

== system cdma2000_lib/cdma2000 Receiver/Rx Channel Structure ==
  note: Performs depuncturing, derepetition, convolutional decoding, encoder tail bits detachment and computes
      | Frame Quality Indicator extraction as described in Figure 3.1.3.1.1.1-15
  note: Rx Channel Structure for
      | Forward Fundamental Channel - Radio Configuration 3
  Modulation Symbols : Inport  LatchInput=off
  Block Deinterleaver : commblkintrlv2/General Block Deinterleaver  elements=interTable
  DePuncture : commsequence2/Insert Zero  insertZeroVector=[1;1;1;1;0]
  Derepeat : commsequence2/Derepeat  N=8  ic=0  mode=Maintain input frame rate
  Encoder Tail Bits : dspsigops/Zero Pad  padSigAt=End  zpadAlong=Columns  padNumOutRowsSpecMethod=User-specified  numOutRows=16 + 6  padNumOutColsSpecMethod=User-specified  numOutCols=1  trunc_flag=None
  Extract FQI : commcrc2/General CRC Syndrome Detector  genPoly=[6 5 2 1 0]  iniStates=[1]  numChecksums=1
  Viterbi Decoder : commcnvcod2/Viterbi Decoder  trellis=poly2trellis(9, [765 671 513 473])  dectype=Unquantized  nsdecb=4  tbdepth=30  opmode=Truncated  reset=off
  Channel Bits : Outport
  FQI : Outport  Port=2
  wires:
  DePuncture/1 -> Derepeat/1
  Derepeat/1 -> Viterbi Decoder/1
  Viterbi Decoder/1 -> Encoder Tail Bits/1
  Modulation Symbols/1 -> Block Deinterleaver/1
  Encoder Tail Bits/1 -> Extract FQI/1
  Extract FQI/2 -> FQI/1
  Extract FQI/1 -> Channel Bits/1
  Block Deinterleaver/1 -> DePuncture/1

== system cdma2000_lib/cdma2000 Receiver/Symbol Demapping ==
  In1 : Inport  LatchInput=off
  Complex to Real-Imag : ComplexToRealImag
  Matrix Concatenation : simulink/Math Operations/Matrix Concatenation  numInports=2  catMethod=Vertical
  Out1 : Outport
  wires:
  Complex to Real-Imag/1 -> Matrix Concatenation/1
  Complex to Real-Imag/2 -> Matrix Concatenation/2
  In1/1 -> Complex to Real-Imag/1
  Matrix Concatenation/1 -> Out1/1

== system cdma2000_lib/cdma2000 Transmitter/Baseband Filtering ==
  note: I and Q components are applied to the I and Q baseband filters separately
      | as described in 3.1.3.1.12
  note: Baseband Filtering
  InData : Inport  LatchInput=off
  Interpolation Filtering : dspmlti3/FIR Interpolation  h=h_k  L=4  framing=Maintain input frame rate  outputBufInitCond=0  roundingMode=Floor  overflowMode=off
  OutData : Outport
  wires:
  InData/1 -> Interpolation Filtering/1
  Interpolation Filtering/1 -> OutData/1

== system cdma2000_lib/cdma2000 Transmitter/Long Code Scrambling ==
  note: Data scrambling for Forward Traffic Channel as described in TIA/EIA/IS-2000.2.A 3.1.3.1.9
  note: Long Code Scrambling
  InData : Inport  LatchInput=off
  Long Code : Inport  Port=2  LatchInput=off
  Buffer : dspbuff3/Buffer  N=2*scrBitRepetition*24  V=0  ic=0
      settings: AttributesFormatString=\n
  DSP Constant1 : dspsrcs4/DSP Constant  Value=longCodeScrOff  SampleMode=Discrete  discreteOutput=Sample-based  continuousOutput=Sample-based  sampTime=20e-3/16  framePeriod=20e-3/16  dataType=Inherit from 'Constant value'  wordLen=16  udDataType=sfix(16)  fracBitsMode=Best precision  numFracBits=15  InterpretAs1D=off  Ts=20e-3/16  FramebasedOutput=off
      settings: AttributesFormatString=\n\n\n\n
  Logical Operator : Logic  Operator=NOT  AllPortsSameDT=off
  Long Code Scrambling : Subsystem  PropExecContextAcrossSSBoundary=on
  Switch1 : Switch  Criteria=u2 > Threshold  Threshold=0.5  SaturateOnIntegerOverflow=on
  Unipolar to Bipolar Converter2 : commutil2/Unipolar to Bipolar Converter  M=2  polarity=Negative
  OutData : Outport
  wires:
  Logical Operator/1 -> Long Code Scrambling/Enable
  Long Code/1 -> Long Code Scrambling/2(longCode)
  Unipolar to Bipolar Converter2/1 -> Long Code Scrambling/1(InData), Switch1/1
  Buffer/1 -> Unipolar to Bipolar Converter2/1
  Switch1/1 -> OutData/1
  Long Code Scrambling/1(OutData) -> Switch1/3
  DSP Constant1/1 -> Logical Operator/1, Switch1/2
  InData/1 -> Buffer/1

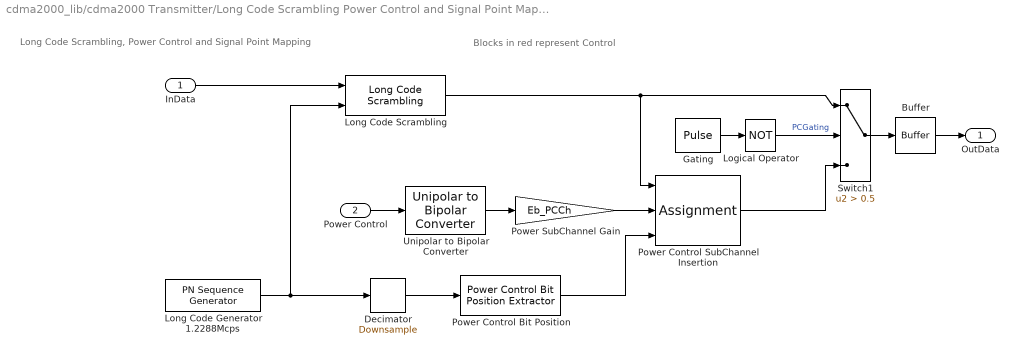
== system cdma2000_lib/cdma2000 Transmitter/Long Code Scrambling Power Control and Signal Point Mapping ==
  note: Long Code Scrambling, Power Control and Signal Point Mapping
  note: Blocks in red represent Control
  InData : Inport  LatchInput=off
  Power Control : Inport  Port=2  LatchInput=off
  Buffer : dspbuff3/Buffer  N=2*scrBitRepetition  V=0  ic=0
  Decimator : dspsigops/Downsample  N=64/2  phase=0  ic=0  smode=Allow multirate  fmode=Maintain input frame rate
      settings: AttributesFormatString=\n
  Gating : DiscretePulseGenerator  Amplitude=powerControlOff  Period=1/gateRate  PhaseDelay=PCGroupInit  SampleTime=20e-3/16
  Logical Operator : Logic  Operator=NOT  AllPortsSameDT=off
  Long Code Scrambling : cdma2000_lib/cdma2000 Transmitter/Long Code Scrambling  SimViewingDevice=off  DataTypeOverride=UseLocalSettings  MinMaxOverflowLogging=UseLocalSettings
      settings: Permissions=ReadWrite  RTWFcnNameOpts=Auto  RTWFileNameOpts=Auto
  Long Code Generator 1.2288Mcps : commseqgen2/PN Sequence Generator  poly=[42 35 33 31 27 26 25 22 21 19 18 17 16 10 7 6 5 3 2 1 0]  ini_sta=[1]  shift=plcMask  Ts=1/1.2288e6  frameBased=on  sampPerFrame=64*24*scrBitRepetition  reset=off
  Power Control Bit Position : cdma2000_lib/cdma2000 Transmitter/Power Control Bit Position Extractor  SimViewingDevice=off  DataTypeOverride=UseLocalSettings  MinMaxOverflowLogging=UseLocalSettings
      settings: Permissions=ReadWrite  RTWFcnNameOpts=Auto  RTWFileNameOpts=Auto
  Power Control SubChannel Insertion : Assignment  ElementSrc=External
  Power SubChannel Gain : Gain  Gain=Eb_PCCh  SaturateOnIntegerOverflow=on
  Switch1 : Switch  Criteria=u2 > Threshold  Threshold=0.5  SaturateOnIntegerOverflow=on
  Unipolar to Bipolar Converter : commutil2/Unipolar to Bipolar Converter  M=2  polarity=Negative
  OutData : Outport
  wires:
  Logical Operator/1 -> Switch1/2  "PCGating"
  Unipolar to Bipolar Converter/1 -> Power SubChannel Gain/1
  InData/1 -> Long Code Scrambling/1
  Power SubChannel Gain/1 -> Power Control SubChannel Insertion/2
  Power Control/1 -> Unipolar to Bipolar Converter/1
  Switch1/1 -> Buffer/1
  Long Code Generator 1.2288Mcps/1 -> Long Code Scrambling/2, Decimator/1
  Power Control SubChannel Insertion/1 -> Switch1/3
  Gating/1 -> Logical Operator/1
  Buffer/1 -> OutData/1
  Power Control Bit Position/1 -> Power Control SubChannel Insertion/3
  Long Code Scrambling/1 -> Switch1/1, Power Control SubChannel Insertion/1
  Decimator/1 -> Power Control Bit Position/1

== system cdma2000_lib/cdma2000 Transmitter/Non-TD Demultiplexer ==
  InData : Inport  LatchInput=off
  Non-TD Demultiplexer : dspindex/Multiport Selector  rowsOrCols=Rows  idxCellArray={1,2}  idxErrMode=Clip Index
      settings: AttributesFormatString=\n
  I1 : Outport
  Q1 : Outport  Port=2
  wires:
  InData/1 -> Non-TD Demultiplexer/1
  Non-TD Demultiplexer/2 -> Q1/1
  Non-TD Demultiplexer/1 -> I1/1

== system cdma2000_lib/cdma2000 Transmitter/Power Control Bit Position Extractor ==
  note: Compute Power Control Bit Position for
      | Power Control subchannel as described in TIA/EIA/IS-2000.2.A  3.1.3.1.10
  note: Power Control Bit Position
      | Extractor
  Decimated Bits : Inport  LatchInput=off
  Bit to Integer Converter : commutil2/Bit to Integer Converter  nbits=length(decPattern)
  DSP Constant3 : dspsrcs4/DSP Constant  Value=[1:numPuncturedSymbols]  SampleMode=Discrete  discreteOutput=Sample-based  continuousOutput=Sample-based  sampTime=1.25e-3  framePeriod=1.25e-3  dataType=Inherit from 'Constant value'  wordLen=16  udDataType=sfix(16)  fracBitsMode=Best precision  numFracBits=15  InterpretAs1D=off  Ts=1.25e-3  FramebasedOutput=off
  Decimator1 : dspindex/Multiport Selector  rowsOrCols=Rows  idxCellArray={decPattern}  idxErrMode=Clip Index
      settings: AttributesFormatString=\n
  Frame Status Conversion1 : dspsigattribs/Frame Status Conversion  growRefPort=off  outframe=Sample-based
  Starting Symbol Position : Gain  Gain=2*scrBitRepetition  SaturateOnIntegerOverflow=on
  Sum : Sum  Inputs=|++  SaturateOnIntegerOverflow=on
  Bits : Outport
  wires:
  Frame Status Conversion1/1 -> Bits/1
  DSP Constant3/1 -> Sum/2
  Sum/1 -> Frame Status Conversion1/1
  Starting Symbol Position/1 -> Sum/1
  Bit to Integer Converter/1 -> Starting Symbol Position/1
  Decimator1/1 -> Bit to Integer Converter/1
  Decimated Bits/1 -> Decimator1/1

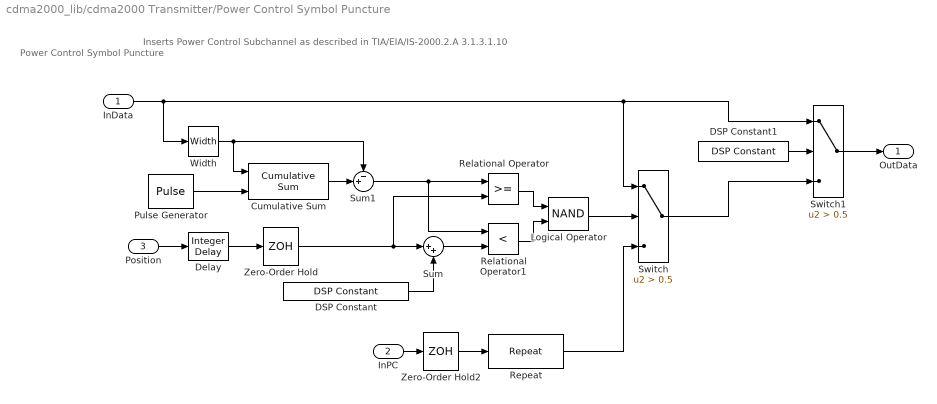
== system cdma2000_lib/cdma2000 Transmitter/Power Control Symbol Puncture ==
  note: Power Control Symbol Puncture
  note: Inserts Power Control Subchannel as described in TIA/EIA/IS-2000.2.A 3.1.3.1.10
  InData : Inport  LatchInput=off
  InPC : Inport  Port=2  LatchInput=off
  Position : Inport  Port=3  LatchInput=off
  Cumulative Sum : dspmathops/Cumulative Sum  dim=Channels (running sum)  reset_popup=Non-zero sample
  DSP Constant : dspsrcs4/DSP Constant  Value=numPuncturedSymbols  SampleMode=Discrete  discreteOutput=Sample-based  continuousOutput=Sample-based  sampTime=symbolTime*scrBitRepetition  framePeriod=symbolTime*scrBitRepetition  dataType=Inherit from 'Constant value'  wordLen=16  udDataType=sfix(16)  fracBitsMode=Best precision  numFracBits=15  InterpretAs1D=off  Ts=symbolTime*scrBitRepetition  FramebasedOutput=off
      settings: AttributesFormatString=\n\n\n\n
  DSP Constant1 : dspsrcs4/DSP Constant  Value=powerControlOff  SampleMode=Discrete  discreteOutput=Sample-based  continuousOutput=Sample-based  sampTime=symbolTime*scrBitRepetition  framePeriod=symbolTime*scrBitRepetition  dataType=Inherit from 'Constant value'  wordLen=16  udDataType=sfix(16)  fracBitsMode=Best precision  numFracBits=15  InterpretAs1D=off  Ts=symbolTime*scrBitRepetition  FramebasedOutput=off
      settings: AttributesFormatString=\n\n\n\n
  Delay : dspobslib/Integer Delay  delay=1  ic=0  reset_popup=None
      settings: AttributesFormatString=\n
  Logical Operator : Logic  Operator=NAND  AllPortsSameDT=off
  Pulse Generator : DiscretePulseGenerator  Period=numSymbPCGroup/(gateRate*2*scrBitRepetition)  PhaseDelay=PCGroupInit  SampleTime=symbolTime*scrBitRepetition
  Relational Operator : RelationalOperator
  Relational Operator1 : RelationalOperator  Operator=<
  Repeat : dspsigops/Repeat  N=2*scrBitRepetition  ic=0  mode=Maintain input frame rate
  Sum : Sum  Inputs=|++  SaturateOnIntegerOverflow=on
  Sum1 : Sum  Inputs=-+|  SaturateOnIntegerOverflow=on
  Switch : Switch  Criteria=u2 > Threshold  Threshold=0.5  SaturateOnIntegerOverflow=on
  Switch1 : Switch  Criteria=u2 > Threshold  Threshold=0.5  SaturateOnIntegerOverflow=on
  Width : Width
  Zero-Order Hold : ZeroOrderHold  SampleTime=symbolTime*scrBitRepetition
  Zero-Order Hold2 : ZeroOrderHold  SampleTime=symbolTime*scrBitRepetition
  OutData : Outport
  wires:
  Position/1 -> Delay/1
  InPC/1 -> Zero-Order Hold2/1
  Repeat/1 -> Switch/3
  InData/1 -> Width/1, Switch/1, Switch1/1
  Width/1 -> Cumulative Sum/1, Sum1/1
  Delay/1 -> Zero-Order Hold/1
  Sum/1 -> Relational Operator1/2
  DSP Constant/1 -> Sum/2
  Zero-Order Hold/1 -> Relational Operator/2, Sum/1
  Relational Operator/1 -> Logical Operator/1
  Relational Operator1/1 -> Logical Operator/2
  Logical Operator/1 -> Switch/2
  Pulse Generator/1 -> Cumulative Sum/2
  Cumulative Sum/1 -> Sum1/2
  Sum1/1 -> Relational Operator/1, Relational Operator1/1
  Zero-Order Hold2/1 -> Repeat/1
  Switch1/1 -> OutData/1
  Switch/1 -> Switch1/3
  DSP Constant1/1 -> Switch1/2
